simulink model "YCrCb_Lab_WithBackgroundRemove_Threshoding"  (R2016a)
settings: Solver=VariableStepAuto  StartTime=0.0  StopTime=10.0  RelTol=1e-3
undefined symbols (not defined in the file): Rec, SDTV
libraries: visionsinks x10, visionconversions x5, visionsources x2
settings Model: Creator=YASARA  LastModifiedBy=YASARA

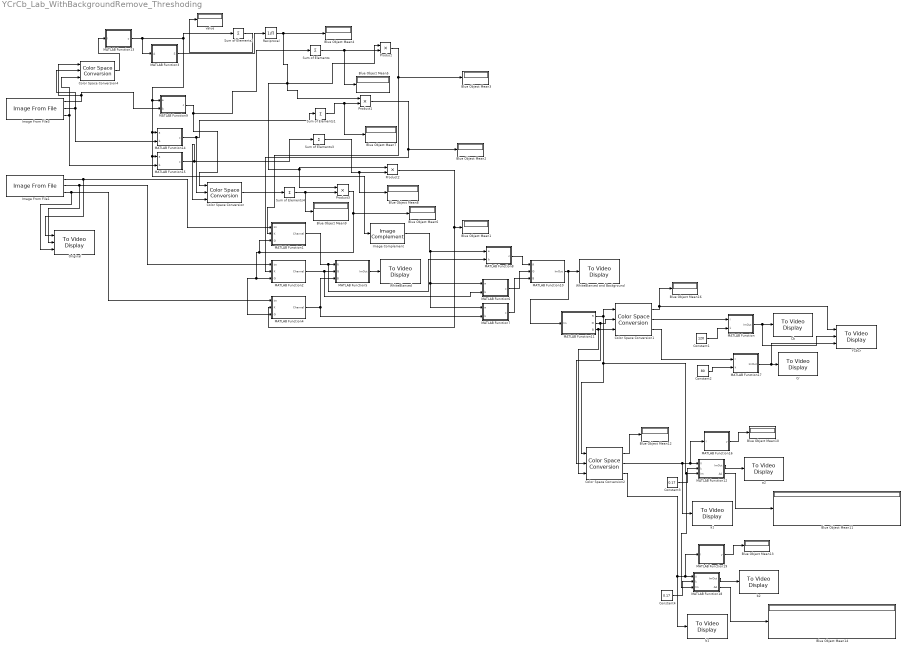
== system YCrCb_Lab_WithBackgroundRemove_Threshoding ==
  Blue Object Mean{1..14,16} (15 alike) : Display
  Cb : visionsinks/To Video Display  windowSizeMode=Normal  openAtMdlStart=on  fullScreen=off  videoWindowX=252  videoWindowY=213  saveWindowSize=off  videoWindowWidth=512  videoWindowHeight=384  inputColorFormat=RGB  inputType=Obsolete  imagePorts=One multidimensional signal  OutputDevice=On-screen video monitor  dataOrg=Column-major  isWindowOpen=off
  Color Space Conversion : visionconversions/Color Space  Conversion  conversion=Obsolete  conversionActive=R'G'B' to intensity  wp_str=D65  rec=Rec. 601 (SDTV)  sys=1125/60/2:1  imagePorts=Separate color signals
  Color Space Conversion1 : visionconversions/Color Space  Conversion  conversion=Obsolete  conversionActive=R'G'B' to Y'CbCr  wp_str=D65  rec=Rec. 601 (SDTV)  sys=1125/60/2:1  imagePorts=Separate color signals
  Color Space Conversion2 : visionconversions/Color Space  Conversion  conversion=Obsolete  conversionActive=sR'G'B' to L*a*b*  wp_str=D65  rec=Rec. 601 (SDTV)  sys=1125/60/2:1  imagePorts=Separate color signals
  Color Space Conversion4 : visionconversions/Color Space  Conversion  conversion=Obsolete  conversionActive=R'G'B' to intensity  wp_str=D65  rec=Rec. 601 (SDTV)  sys=1125/60/2:1  imagePorts=Separate color signals
  Constant1 : Constant  Value=120
  Constant2 : Constant  Value=80
  Constant3 : Constant  Value=0.17  OutDataTypeStr=double
  Constant4 : Constant  Value=0.17  OutDataTypeStr=double
  Cr : visionsinks/To Video Display  windowSizeMode=Normal  openAtMdlStart=on  fullScreen=off  videoWindowX=252  videoWindowY=213  saveWindowSize=off  videoWindowWidth=512  videoWindowHeight=384  inputColorFormat=RGB  inputType=Obsolete  imagePorts=One multidimensional signal  OutputDevice=On-screen video monitor  dataOrg=Column-major  isWindowOpen=off
  Image Complement : visionconversions/Image Complement
  Image From File1 : visionsources/Image From File  Tag=vipblks_nd  FileName=C:\Users\YASARA\Desktop\FYPReview\New folder\Stem_Leaf\DSC_1206.JPG  imagePorts=Separate color signals  Ts=1  ImageDataType=uint8  Signed=on  WordLength=16  sdImageDataType=uint(8)  FractionLengthMode=User-defined  FractionLength=15  OutPortLabels=R|G|B
  Image From File3 : visionsources/Image From File  Tag=vipblks_nd  FileName=C:\Users\YASARA\Desktop\FYPReview\New folder\Stem_Leaf\DSC_1206.JPG  imagePorts=Separate color signals  Ts=1  ImageDataType=double  Signed=on  WordLength=16  sdImageDataType=uint(8)  FractionLengthMode=User-defined  FractionLength=15  OutPortLabels=R|G|B
  MATLAB Function : MATLAB Function  TreatAsAtomicUnit=on
  MATLAB Function1 : MATLAB Function  TreatAsAtomicUnit=on
  MATLAB Function10 : MATLAB Function  TreatAsAtomicUnit=on
  MATLAB Function11 : MATLAB Function  TreatAsAtomicUnit=on
  MATLAB Function12 : MATLAB Function  TreatAsAtomicUnit=on
  MATLAB Function13 : MATLAB Function  TreatAsAtomicUnit=on
  MATLAB Function14 : MATLAB Function  TreatAsAtomicUnit=on
  MATLAB Function15 : MATLAB Function  TreatAsAtomicUnit=on
  MATLAB Function16 : MATLAB Function  TreatAsAtomicUnit=on
  MATLAB Function17 : MATLAB Function  TreatAsAtomicUnit=on
  MATLAB Function18 : MATLAB Function  TreatAsAtomicUnit=on
  MATLAB Function19 : MATLAB Function  TreatAsAtomicUnit=on
  MATLAB Function2 : MATLAB Function  TreatAsAtomicUnit=on
  MATLAB Function3 : MATLAB Function  TreatAsAtomicUnit=on
  MATLAB Function4 : MATLAB Function  TreatAsAtomicUnit=on
  MATLAB Function5 : MATLAB Function  TreatAsAtomicUnit=on
  MATLAB Function6 : MATLAB Function  TreatAsAtomicUnit=on
  MATLAB Function7 : MATLAB Function  TreatAsAtomicUnit=on
  MATLAB Function8 : MATLAB Function  TreatAsAtomicUnit=on
  MATLAB Function9 : MATLAB Function  TreatAsAtomicUnit=on
  Original : visionsinks/To Video Display  windowSizeMode=Normal  openAtMdlStart=on  fullScreen=off  videoWindowX=252  videoWindowY=213  saveWindowSize=off  videoWindowWidth=512  videoWindowHeight=384  inputColorFormat=RGB  inputType=Obsolete  imagePorts=Separate color signals  OutputDevice=On-screen video monitor  dataOrg=Column-major  isWindowOpen=off
  Product{,1..3} (4 alike) : Product  OutDataTypeStr=uint8
  Reciprocal : Product  Inputs=/  OutDataTypeStr=double  SaturateOnIntegerOverflow=on  RndMeth=Zero
  Sum of Elements{,1..4} (5 alike) : Sum  Inputs=+
  WhiteBlanced : visionsinks/To Video Display  windowSizeMode=Normal  openAtMdlStart=on  fullScreen=off  videoWindowX=252  videoWindowY=213  saveWindowSize=off  videoWindowWidth=512  videoWindowHeight=384  inputColorFormat=RGB  inputType=Obsolete  imagePorts=One multidimensional signal  OutputDevice=On-screen video monitor  dataOrg=Column-major  isWindowOpen=off
  WhiteBlanced and Background : visionsinks/To Video Display  windowSizeMode=Normal  openAtMdlStart=on  fullScreen=off  videoWindowX=252  videoWindowY=213  saveWindowSize=off  videoWindowWidth=512  videoWindowHeight=384  inputColorFormat=RGB  inputType=Obsolete  imagePorts=One multidimensional signal  OutputDevice=On-screen video monitor  dataOrg=Column-major  isWindowOpen=off
  YCbCr : visionsinks/To Video Display  windowSizeMode=Normal  openAtMdlStart=on  fullScreen=off  videoWindowX=252  videoWindowY=213  saveWindowSize=off  videoWindowWidth=512  videoWindowHeight=384  inputColorFormat=RGB  inputType=Obsolete  imagePorts=Separate color signals  OutputDevice=On-screen video monitor  dataOrg=Column-major  isWindowOpen=off
  a1 : visionsinks/To Video Display  windowSizeMode=Normal  openAtMdlStart=on  fullScreen=off  videoWindowX=252  videoWindowY=213  saveWindowSize=off  videoWindowWidth=512  videoWindowHeight=384  inputColorFormat=RGB  inputType=Obsolete  imagePorts=One multidimensional signal  OutputDevice=On-screen video monitor  dataOrg=Column-major  isWindowOpen=off
  a2 : visionsinks/To Video Display  windowSizeMode=Normal  openAtMdlStart=on  fullScreen=off  videoWindowX=252  videoWindowY=213  saveWindowSize=off  videoWindowWidth=512  videoWindowHeight=384  inputColorFormat=RGB  inputType=Obsolete  imagePorts=One multidimensional signal  OutputDevice=On-screen video monitor  dataOrg=Column-major  isWindowOpen=off
  b1 : visionsinks/To Video Display  windowSizeMode=Normal  openAtMdlStart=on  fullScreen=off  videoWindowX=252  videoWindowY=213  saveWindowSize=off  videoWindowWidth=512  videoWindowHeight=384  inputColorFormat=RGB  inputType=Obsolete  imagePorts=One multidimensional signal  OutputDevice=On-screen video monitor  dataOrg=Column-major  isWindowOpen=off
  b2 : visionsinks/To Video Display  windowSizeMode=Normal  openAtMdlStart=on  fullScreen=off  videoWindowX=252  videoWindowY=213  saveWindowSize=off  videoWindowWidth=512  videoWindowHeight=384  inputColorFormat=RGB  inputType=Obsolete  imagePorts=One multidimensional signal  OutputDevice=On-screen video monitor  dataOrg=Column-major  isWindowOpen=off
  value : Display
  wires:
  Color Space Conversion4/1 -> MATLAB Function13/1(I)
  MATLAB Function9/1(c) -> Color Space Conversion/1, Sum of Elements/1
  MATLAB Function14/1(c) -> Sum of Elements1/1, Color Space Conversion/2
  MATLAB Function15/1(c) -> Sum of Elements3/1, Color Space Conversion/3
  Reciprocal/1 -> Product1/1, Product3/1, Product2/1, Product/1, Blue Object Mean4/1
  MATLAB Function13/1(y) -> MATLAB Function3/1(A), Image Complement/1, MATLAB Function15/1(a), MATLAB Function14/1(a), MATLAB Function9/1(a), Sum of Elements2/1
  Image From File3/1 -> MATLAB Function9/2(b), Color Space Conversion4/1
  Image From File3/2 -> MATLAB Function14/2(b), Color Space Conversion4/2
  Image From File3/3 -> Color Space Conversion4/3, MATLAB Function15/2(b)
  Image From File1/2 -> Original/2, MATLAB Function2/1(Im)
  Image From File1/3 -> Original/3, MATLAB Function4/1(Im)
  Product/1 -> MATLAB Function1/2(K), Blue Object Mean3/1
  Product1/1 -> Blue Object Mean2/1, MATLAB Function2/2(K)
  Product2/1 -> MATLAB Function4/2(K), Blue Object Mean1/1
  Color Space Conversion/1 -> Sum of Elements4/1
  Sum of Elements/1 -> Blue Object Mean5/1, Product/2
  Product3/1 -> Blue Object Mean6/1, MATLAB Function4/3(G), MATLAB Function2/3(G), MATLAB Function1/3(G)
  Sum of Elements1/1 -> Blue Object Mean7/1, Product1/2
  Sum of Elements3/1 -> Blue Object Mean8/1, Product2/2
  Sum of Elements4/1 -> Blue Object Mean9/1, Product3/2
  Sum of Elements2/1 -> value/1
  MATLAB Function3/1(S) -> Reciprocal/1
  MATLAB Function2/1(Channel) -> MATLAB Function6/2(b), MATLAB Function5/2(G)
  MATLAB Function4/1(Channel) -> MATLAB Function5/3(B), MATLAB Function7/2(b)
  MATLAB Function5/1(ImOut) -> WhiteBlanced/1
  MATLAB Function1/1(Channel) -> MATLAB Function8/2(b), MATLAB Function5/1(R)
  Image From File1/1 -> Original/1, MATLAB Function1/1(Im)
  Image Complement/1 -> MATLAB Function7/1(a), MATLAB Function6/1(a), MATLAB Function8/1(a)
  MATLAB Function10/1(ImOut) -> MATLAB Function11/1(Im), WhiteBlanced and Background/1
  MATLAB Function8/1(c) -> MATLAB Function10/1(R)
  MATLAB Function6/1(c) -> MATLAB Function10/2(G)
  MATLAB Function7/1(c) -> MATLAB Function10/3(B)
  Color Space Conversion1/1 -> Blue Object Mean16/1, YCbCr/1
  Color Space Conversion1/2 -> MATLAB Function/1(I)
  Constant1/1 -> MATLAB Function/2(k)
  MATLAB Function/1(ImOut) -> YCbCr/2, Cb/1
  Color Space Conversion1/3 -> MATLAB Function17/1(I)
  Constant2/1 -> MATLAB Function17/2(k)
  MATLAB Function17/1(ImOut) -> YCbCr/3, Cr/1
  MATLAB Function11/2(G) -> Color Space Conversion2/2, Color Space Conversion1/2
  Color Space Conversion2/1 -> Blue Object Mean12/1
  Color Space Conversion2/2 -> a1/1, MATLAB Function16/1(I), MATLAB Function12/1(II)
  Constant3/1 -> MATLAB Function12/2(k)
  MATLAB Function12/1(ImOut) -> a2/1
  MATLAB Function16/1(y) -> Blue Object Mean10/1
  MATLAB Function12/2(AA) -> Blue Object Mean11/1
  MATLAB Function11/3(B) -> Color Space Conversion2/3, Color Space Conversion1/3
  MATLAB Function11/1(R) -> Color Space Conversion2/1, MATLAB Function18/3(Im), MATLAB Function12/3(Im), Color Space Conversion1/1
  Color Space Conversion2/3 -> b1/1, MATLAB Function19/1(I), MATLAB Function18/1(II)
  Constant4/1 -> MATLAB Function18/2(k)
  MATLAB Function18/1(ImOut) -> b2/1
  MATLAB Function19/1(y) -> Blue Object Mean13/1
  MATLAB Function18/2(AA) -> Blue Object Mean14/1

== matlab function YCrCb_Lab_WithBackgroundRemove_Threshoding/MATLAB Function1 ==
  data: Im input; K input; Channel output; G input
function Channel = fcn(Im,K,G)
Channel = uint8(double(Im) *double(G)/double(K));
return

== matlab function YCrCb_Lab_WithBackgroundRemove_Threshoding/MATLAB Function2 ==
  data: Im input; K input; Channel output; G input
function Channel = fcn(Im,K,G)
Channel = uint8(double(Im) *double(G)/double(K));
return

== matlab function YCrCb_Lab_WithBackgroundRemove_Threshoding/MATLAB Function3 ==
  data: A input; S output
function S = fcn(A)
%#codegen
S = sum(A(:))/100;

== matlab function YCrCb_Lab_WithBackgroundRemove_Threshoding/MATLAB Function4 ==
  data: Im input; K input; Channel output; G input
function Channel = fcn(Im,K,G)
Channel = uint8(double(Im) *double(G)/double(K));
return

== matlab function YCrCb_Lab_WithBackgroundRemove_Threshoding/MATLAB Function5 ==
  data: R input; G input; B input; ImOut output
function ImOut = fcn(R,G,B)
ImOut = cat(3, R, G, B);
return

== matlab function YCrCb_Lab_WithBackgroundRemove_Threshoding/MATLAB Function6 ==
  data: a input; b input; c output
function c = fcn(a,b)
%#codegen
%c=logical(a).*double(b);
c=uint8(a).*uint8(b);

== matlab function YCrCb_Lab_WithBackgroundRemove_Threshoding/MATLAB Function7 ==
  data: a input; b input; c output
function c = fcn(a,b)
%#codegen
%c=logical(a).*double(b);
c=uint8(a).*uint8(b);

== matlab function YCrCb_Lab_WithBackgroundRemove_Threshoding/MATLAB Function8 ==
  data: a input; b input; c output
function c = fcn(a,b)
%#codegen
c=uint8(a).*uint8(b);
%c=uint8(b);

== matlab function YCrCb_Lab_WithBackgroundRemove_Threshoding/MATLAB Function10 ==
  data: R input; G input; B input; ImOut output
function ImOut = fcn(R,G,B)
ImOut = cat(3, R, G, B);
return

== matlab function YCrCb_Lab_WithBackgroundRemove_Threshoding/MATLAB Function14 ==
  data: a input; b input; c output
function c = fcn(a,b)
%#codegen
c=a.*b;
return

== matlab function YCrCb_Lab_WithBackgroundRemove_Threshoding/MATLAB Function11 ==
  data: Im input; R output; G output; B output
function [R,G,B] = fcn(Im)
R = double(Im(:,:,1));
G = double(Im(:,:,2));
B = double(Im(:,:,3));
return

== matlab function YCrCb_Lab_WithBackgroundRemove_Threshoding/MATLAB Function12 ==
  data: II input; ImOut output; k input; Im input; AA output
function [ImOut,AA] = fcn(II,k,Im)
I=double(Im);
coder.extrinsic('graythresh');
coder.extrinsic('im2bw');
level = graythresh(I);
BW = im2bw(I,level);
L=double(I);
coder.extrinsic('bwlabeln');
NUM=1;
BW2=imcomplement(BW);
[L, NUM] = bwlabeln(BW2);
area=1;
n=1;
R1=double(II);
AA=double(zeros(100,1));
i=1;
for n=1:NUM
    [r, c] = find(L==n);
    %if (max(c)~= min(c))&&(max(r)~= min(r))
    if ((max(c)-min(c))>50)&&((max(r)-min(r))>50)
        t=R1(L==n);
        AA(i)=double(mean(t(:)));         
        if (AA(i)>k)
           R1(L==n)=0; 
           
        end
        i=i+1;
    end
end;
ImOut=R1;

== matlab function YCrCb_Lab_WithBackgroundRemove_Threshoding/MATLAB Function16 ==
  data: I input; y output
function y = fcn(I)
y=mean(I(:));

== matlab function YCrCb_Lab_WithBackgroundRemove_Threshoding/MATLAB Function13 ==
  data: I input; y output
function y = fcn(I)
%#codegen
y=I;
 coder.extrinsic('graythresh');
level = graythresh(I);
BW = double(im2bw(I,level));
y = BW;

== matlab function YCrCb_Lab_WithBackgroundRemove_Threshoding/MATLAB Function15 ==
  data: a input; b input; c output
function c = fcn(a,b)
%#codegen
c=a.*b;
return

== matlab function YCrCb_Lab_WithBackgroundRemove_Threshoding/MATLAB Function9 ==
  data: a input; b input; c output
function c = fcn(a,b)
%#codegen
c=a.*b;
return

== matlab function YCrCb_Lab_WithBackgroundRemove_Threshoding/MATLAB Function ==
  data: I input; ImOut output; k input
function ImOut = fcn(I,k)
coder.extrinsic('graythresh');
coder.extrinsic('im2bw');
level = graythresh(I);
BW = im2bw(I,level);
L=double(I);
coder.extrinsic('bwlabeln');
NUM=1;
BW2=imcomplement(BW);
[L, NUM] = bwlabeln(BW2);
area=1;
n=1;
R1=I;
AA=(zeros(8,1));
i=1;
for n=1:NUM
    [r, c] = find(L==n);
    %if (max(c)~= min(c))&&(max(r)~= min(r))
    if ((max(c)-min(c))>50)&&((max(r)-min(r))>50)
        t=R1(L==n);
        AA(i)=mean(t(:));         
        if (AA(i)>k)
           R1(L==n)=0; 
           
        end
        i=i+1;
    end
end
II=I;
II=R1;
ImOut=II;

== matlab function YCrCb_Lab_WithBackgroundRemove_Threshoding/MATLAB Function17 ==
  data: I input; ImOut output; k input
function ImOut = fcn(I,k)
coder.extrinsic('graythresh');
coder.extrinsic('im2bw');
level = graythresh(I);
BW = im2bw(I,level);
L=double(I);
coder.extrinsic('bwlabeln');
NUM=1;
BW2=imcomplement(BW);
[L, NUM] = bwlabeln(BW2);
area=1;
n=1;
R1=I;
AA=(zeros(8,1));
i=1;
for n=1:NUM
    [r, c] = find(L==n);
    %if (max(c)~= min(c))&&(max(r)~= min(r))
    if ((max(c)-min(c))>50)&&((max(r)-min(r))>50)
        t=R1(L==n);
        AA(i)=mean(t(:));         
        if (AA(i)>k)
           R1(L==n)=0; 
           
        end
        i=i+1;
    end
end
II=I;
II=R1;
ImOut=II;

== matlab function YCrCb_Lab_WithBackgroundRemove_Threshoding/MATLAB Function18 ==
  data: II input; ImOut output; k input; Im input; AA output
function [ImOut,AA] = fcn(II,k,Im)
I=Im;
coder.extrinsic('graythresh');
coder.extrinsic('im2bw');
level = graythresh(I);
BW = im2bw(I,level);
L=double(I);
coder.extrinsic('bwlabeln');
NUM=1;
BW2=imcomplement(BW);
[L, NUM] = bwlabeln(BW2);
area=1;
n=1;
R1=double(II);
AA=double(zeros(100,1));
i=1;
for n=1:NUM
    [r, c] = find(L==n);
    %if (max(c)~= min(c))&&(max(r)~= min(r))
    if ((max(c)-min(c))>50)&&((max(r)-min(r))>50)
        t=R1(L==n);
        AA(i)=mean(t(:));         
        if (AA(i)>k)
           R1(L==n)=0; 
           
        end
        i=i+1;
    end
end;
ImOut=R1;

== matlab function YCrCb_Lab_WithBackgroundRemove_Threshoding/MATLAB Function19 ==
  data: I input; y output
function y = fcn(I)
y=mean(I(:));
